simulink model "v3_sim_sf_with_integral_action_sigma_r"  (R2023b)
settings: Solver=VariableStepAuto  StartTime=0.0  StopTime=30  RelTol=1e-3
libraries: simulink x2
settings Model: Creator=kiraa  LastModifiedBy=kiraa

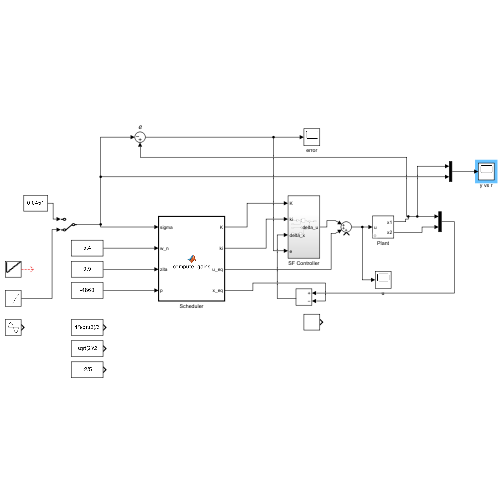
[thumbnail: Simulink's stored preview of the top-level diagram]
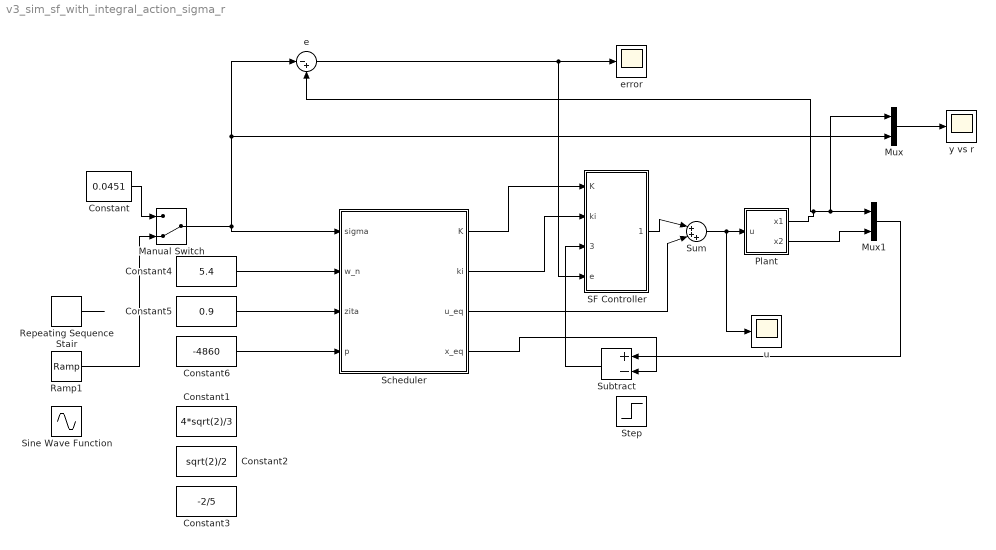
== system v3_sim_sf_with_integral_action_sigma_r ==
  Constant : Constant  Value=0.0451
  Constant1 : Constant  Value=4*sqrt(2)/3
  Constant2 : Constant  Value=sqrt(2)/2
  Constant3 : Constant  Value=-2/5
  Constant4 : Constant  Value=5.4
  Constant5 : Constant  Value=0.9
  Constant6 : Constant  Value=-4860
  Manual Switch : ManualSwitch  CurrentSetting=0
  Mux : Mux  Inputs=2
  Mux1 : Mux  Inputs=2
  Plant : Subsystem  mask{x1_0=0.1, x2_0=0}
      mask prompts: x1_0 "x1(0) [g/l]"; x2_0 "x2(0) [min^-1]"
  Ramp1 : simulink/Sources/Ramp  slope=-0.0005  start=0  InitialOutput=0.1
  Repeating Sequence Stair : simulink/Sources/Repeating Sequence Stair  OutValues=[0.1 0.2 0.3 0.4 0.5 0.6 0.7 0.8 0.9].'  tsamp=20  OutMin=[]  OutMax=[]  OutDataTypeStr=double  OutputDataTypeScalingMode=double  OutDataType=fixdt(0,8)  ConRadixGroup=Best Precision: Vector-wise  OutScaling=2^-12
  SF Controller : Subsystem
  Scheduler : MATLAB Function  TreatAsAtomicUnit=on
  Sine Wave Function : Sin  Amplitude=0.02  Bias=0.05  Frequency=0.1  SampleTime=0
  Step : Step  Time=15  After=50  SampleTime=0
  Subtract : Sum  Inputs=+-
  Sum : Sum  Inputs=|+++
  e : Sum  Inputs=|-+
  error : Scope
  u : Scope
  y vs r : Scope
  wires:
  Plant/1(x1) -> Mux1/1, Mux/1, e/2
  Mux/1 -> y vs r/1
  Constant/1 -> Manual Switch/1
  Manual Switch/1 -> Mux/2, e/1, Scheduler/1(sigma)
  e/1 -> SF Controller/4(e), error/1
  Scheduler/1(K) -> SF Controller/1(K)
  Plant/2(x2) -> Mux1/2
  Constant4/1 -> Scheduler/2(w_n)
  Constant5/1 -> Scheduler/3(zita)
  Scheduler/2(ki) -> SF Controller/2(ki)
  Scheduler/4(x_eq) -> Subtract/2
  Mux1/1 -> Subtract/1
  Subtract/1 -> SF Controller/3(delta_x)
  Sum/1 -> u/1, Plant/1(u)
  SF Controller/1(delta_u) -> Sum/1
  Scheduler/3(u_eq) -> Sum/2
  Repeating Sequence Stair/1 -> ?
  Constant6/1 -> Scheduler/4(p)
  Ramp1/1 -> Manual Switch/2

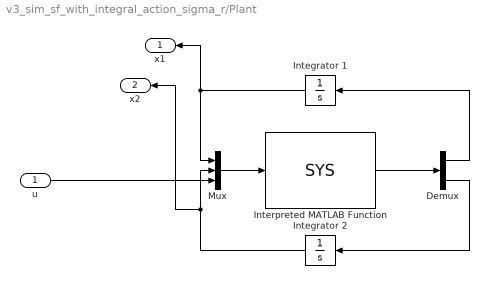
== system v3_sim_sf_with_integral_action_sigma_r/Plant ==
  u : Inport
  Demux : Demux  Outputs=2
  Integrator 1 : Integrator  InitialCondition=x1_0
  Integrator 2 : Integrator  InitialCondition=x2_0
  Interpreted MATLAB Function : MATLABFcn  MATLABFcn=SYS  OutputDimensions=2
  Mux : Mux  Inputs=3
  x1 : Outport
  x2 : Outport  Port=2
  wires:
  Integrator 1/1 -> x1/1, Mux/1
  Demux/1 -> Integrator 1/1
  Mux/1 -> Interpreted MATLAB Function/1
  Integrator 2/1 -> x2/1, Mux/2
  Interpreted MATLAB Function/1 -> Demux/1
  Demux/2 -> Integrator 2/1
  u/1 -> Mux/3

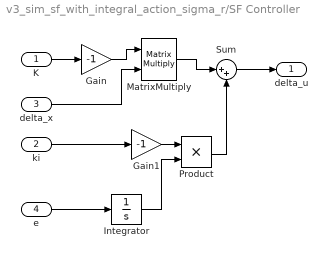
== system v3_sim_sf_with_integral_action_sigma_r/SF Controller ==
  K : Inport
  ki : Inport  Port=2
  delta_x : Inport  Port=3
  e : Inport  Port=4
  Gain : Gain  Gain=-1
  Gain1 : Gain  Gain=-1
  Integrator : Integrator
  MatrixMultiply : Product  Multiplication=Matrix(*)
  Product : Product
  Sum : Sum  Inputs=|++
  delta_u : Outport
  wires:
  K/1 -> Gain/1
  Gain/1 -> MatrixMultiply/1
  MatrixMultiply/1 -> Sum/1
  delta_x/1 -> MatrixMultiply/2
  e/1 -> Integrator/1
  Sum/1 -> delta_u/1
  Integrator/1 -> Product/2
  Product/1 -> Sum/2
  ki/1 -> Gain1/1
  Gain1/1 -> Product/1

== matlab function v3_sim_sf_with_integral_action_sigma_r/Scheduler ==
  data: sigma input; K output; ki output; w_n input; zita input; u_eq output; x_eq output; p input
function [K,ki,u_eq,x_eq] = compute_gains(sigma, w_n, zita,p)

    k1 = -(625*(20769187434139310514121985316880384*sigma^2*w_n^2 - 41538374868278621028243970633760768*p*zita*sigma^2*w_n - 608412576695676974541561223184384*zita*sigma*w_n + 304206288347838487270780611592192*p*sigma + 4455709505430790413433498137721))/(125913198819469569991864535983587328*sigma^3);
 

    k2 = -(2819253366733930496*sigma + 90071992547409920000*p*sigma - 180143985094819840000*sigma*w_n*zita + 1319284474841913125)/(873698327709876224*sigma);
 
    ki = (10000*p*w_n^2)/(97*sigma);
    
    K = [k1 k2];
    x1_eq = sigma;
    x2_eq = -(1360087087465889792*sigma - 1319284474841913125)/(90071992547409920000*sigma);
 
    u_eq = -(399496308545527218176*sigma - 412936040625518808125)/(8736983277098762240000*sigma);
    x_eq = [x1_eq;x2_eq];
end
